simulink model "compliance_control"  (R2021b)
settings: Solver=VariableStepAuto  StartTime=0.0  StopTime=10  RelTol=1e-3
undefined symbols (not defined in the file): dqi, g_q, K, KD, KP, myRobot, qf, qi, qr, xd, xr
libraries: vrlib x1
settings Model: Creator=simon  LastModifiedBy=miche
settings SolverCC: AlgebraicLoopSolver=TrustRegion
settings DebuggingCC: SFMachineParentedDataDiag=warning

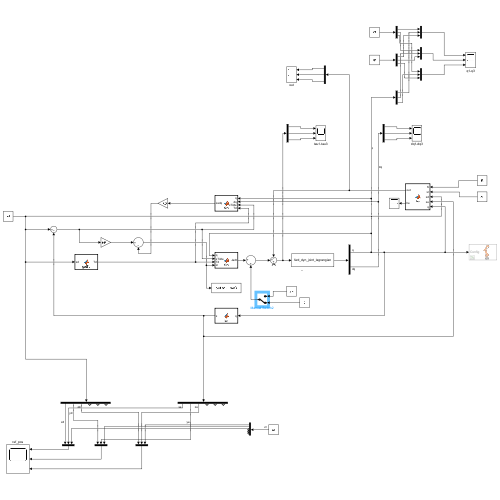
[thumbnail: Simulink's stored preview of the top-level diagram]
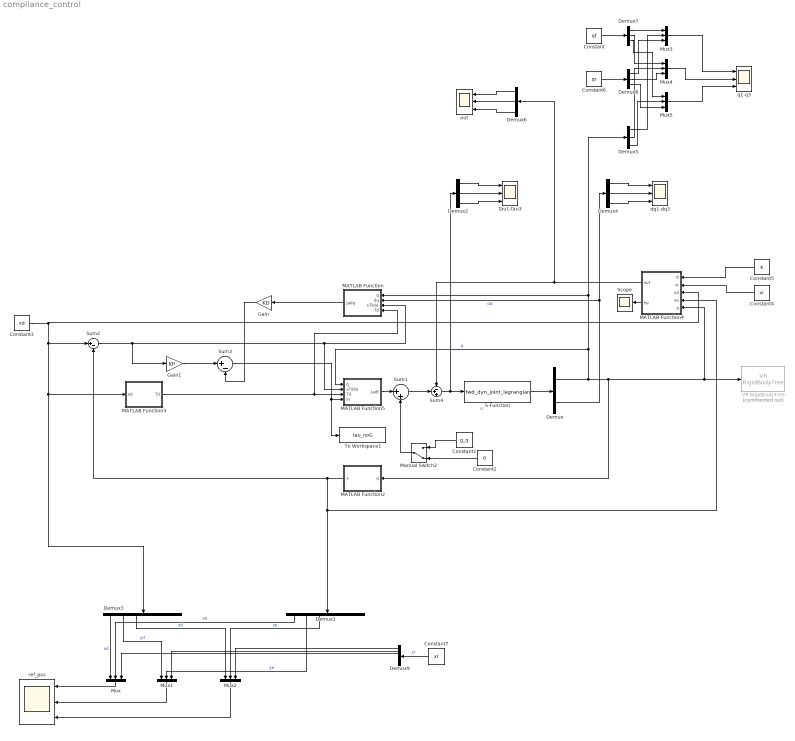
== system compliance_control ==
  note: u
  Constant : Constant  Value=qf
  Constant1 : Constant  Value=g_q
  Constant2 : Constant  Value=0
  Constant3 : Constant  Value=xd
  Constant4 : Constant  Value=xr
  Constant5 : Constant  Value=K
  Constant6 : Constant  Value=qr
  Constant7 : Constant  Value=xr
  Demux : Demux  Outputs=2
  Demux1 : Demux  Outputs=6
  Demux{2,4..6} (4 alike) : Demux  Outputs=myRobot.N
  Demux3 : Demux  Outputs=6
  Demux7 : Demux  Outputs=3
  Demux8 : Demux  Outputs=3
  Demux9 : Demux  Outputs=6
  Gain : Gain  Gain=KD
  Gain1 : Gain  Gain=KP
  MATLAB Function : MATLAB Function  TreatAsAtomicUnit=on
  MATLAB Function2 : MATLAB Function  TreatAsAtomicUnit=on
  MATLAB Function3 : MATLAB Function  TreatAsAtomicUnit=on
  MATLAB Function4 : MATLAB Function  TreatAsAtomicUnit=on
  MATLAB Function5 : MATLAB Function  TreatAsAtomicUnit=on
  Manual Switch2 : ManualSwitch  CurrentSetting=0
  Mux{,1..5} (6 alike) : Mux  Inputs=3
  S-Function : S-Function  FunctionName=fwd_dyn_joint_lagrangian  Parameters=myRobot,qi,dqi  SFunctionDeploymentMode=off  EnableBusSupport=off
  Scope : Scope
  Sum1 : Sum  Inputs=|++
  Sum2 : Sum  Inputs=|+-
  Sum3 : Sum  Inputs=|+-
  Sum4 : Sum  Inputs=-++
  To Workspace1 : ToWorkspace  VariableName=tau_noG  SaveFormat=Timeseries  SampleTime=-1
  VR RigidBodyTree : vrlib/VR RigidBodyTree  Commented=on  RBT=rbt  useRBT=on  Ts=-1  ForceViewerOpen=on
      settings: SourceProductBaseCode=SL
  dq1-dq3 : Scope  NumInputPorts=3
  out : Scope  NumInputPorts=3
  q1-q3 : Scope  NumInputPorts=3
  ref_pos : Scope  NumInputPorts=3
  tau1-tau3 : Scope  NumInputPorts=3
  wires:
  Constant1/1 -> Manual Switch2/1
  Constant2/1 -> Manual Switch2/2
  Mux2/1 -> ref_pos/3
  Demux3/2 -> Mux1/1  "yd"
  Mux1/1 -> ref_pos/2
  Demux3/1 -> Mux/1  "xd"
  Mux/1 -> ref_pos/1
  Sum4/1 -> S-Function/1, Demux2/1
  Demux2/3 -> tau1-tau3/3
  Constant3/1 -> MATLAB Function4/3(xd), Demux3/1, MATLAB Function3/1(xd), Sum2/1
  Manual Switch2/1 -> Sum1/2
  Sum1/1 -> Sum4/2
  Demux4/1 -> dq1-dq3/1
  Demux4/3 -> dq1-dq3/3
  Sum2/1 -> MATLAB Function/3(xTilde), MATLAB Function5/2(xTilde), Gain1/1
  Demux4/2 -> dq1-dq3/2
  Gain1/1 -> Sum3/1
  Demux1/1 -> Mux/2  "xe"
  Sum3/1 -> To Workspace1/1, MATLAB Function5/4(in)
  Demux3/3 -> Mux2/1  "zd"
  S-Function/1 -> Demux/1
  Demux/2 -> MATLAB Function/2(dq), Demux4/1  "dq"
  Gain/1 -> Sum3/2
  Demux1/2 -> Mux1/2  "ye"
  Demux2/1 -> tau1-tau3/1
  Demux2/2 -> tau1-tau3/2
  MATLAB Function/1(Jadq) -> Gain/1
  MATLAB Function5/1(Jadt) -> Sum1/1
  MATLAB Function2/1(x) -> MATLAB Function4/4(xe), Demux1/1, Sum2/2
  MATLAB Function3/1(Td) -> MATLAB Function5/3(Td), MATLAB Function/4(Td)
  MATLAB Function4/1(out) -> Demux6/1, Sum4/1
  Constant4/1 -> MATLAB Function4/2(xr)
  Constant5/1 -> MATLAB Function4/1(K)
  MATLAB Function4/2(he) -> Scope/1
  Demux5/3 -> Mux5/2
  Demux5/1 -> Mux3/2
  Demux5/2 -> Mux4/2
  Demux/1 -> MATLAB Function2/1(q), VR RigidBodyTree/1, MATLAB Function4/5(q), MATLAB Function/1(q), Demux5/1, MATLAB Function5/1(q)  "q"
  Demux1/3 -> Mux2/2  "ze"
  Demux6/2 -> out/2
  Demux6/1 -> out/1
  Demux6/3 -> out/3
  Constant/1 -> Demux7/1
  Constant6/1 -> Demux8/1
  Demux7/1 -> Mux3/1
  Demux8/1 -> Mux3/3
  Mux3/1 -> q1-q3/1
  Demux7/2 -> Mux4/1
  Demux8/2 -> Mux4/3
  Mux4/1 -> q1-q3/2
  Demux7/3 -> Mux5/1
  Demux8/3 -> Mux5/3
  Mux5/1 -> q1-q3/3
  Constant7/1 -> Demux9/1  "zr"
  Demux9/3 -> Mux/3
  Demux9/2 -> Mux1/3
  Demux9/1 -> Mux2/3

== matlab function compliance_control/MATLAB Function ==
  data: q input size=3; Jadq output size=6; dq input; xTilde input; Td input
function Jadq = fcn(q, dq,xTilde, Td)

Jadq =getJad(q,xTilde,Td)*dq;

== matlab function compliance_control/MATLAB Function2 ==
  data: q input; x output
function x = fcn(q)
x = getK(q);

== matlab function compliance_control/MATLAB Function3 ==
  data: xd input; Td output
function Td = getTd(xd)
%xd(4:6) are the phi angle
Rd = eul2rotm(xd(4:6)','ZYZ');
%xd(1:3) is the position 
t = xd(1:3);
Td = [Rd t
    zeros(1,3) 1];

== matlab function compliance_control/MATLAB Function4 ==
  data: K input; out output size=3; xr input; xd input; xe input; q input; he output
function [out, he]= he(K, xr, xd, xe, q)
%consider the interaction only in z direction
q1 = q(1);
q3 = q(3);
a1 = 0.4;
a3 = 0.24;

% if the end effector touch the environment 
if xe(3) < xr(3)
    dxrd = xd-xr;
    dxed = xd-xe;
    dxre = dxrd-dxed;
    %The interaction force between the end-effector and the environment is
    he = K*dxre;
else
    he = zeros(6,1);
end

Jtransp = [
[- a3*sin(q1 + q3) - a1*sin(q1), a3*cos(q1 + q3) + a1*cos(q1), 0, 0, 0, 1]
[                             0,                            0, 1, 0, 0, 0]
[              -a3*sin(q1 + q3),              a3*cos(q1 + q3), 0, 0, 0, 1]
];
%If there is interaction with the environment (hde != 0) the equilibrium will be at the pose
%Jtransp(q)* hde
out = Jtransp*he;

== matlab function compliance_control/MATLAB Function5 ==
  data: q input size=3; Jadt output size=3; xTilde input; Td input; in input
function Jadt = fcn(q, xTilde, Td, in)

Jadt =getJad(q,xTilde,Td)'*in;
